simulink model "chap4_3sim"  (Simulink 5.0)
settings: Solver=ode45  StartTime=0.0  StopTime=20  RelTol=1e-5
settings Model: LastModifiedBy=Administrator  ExtModeTrigMode=oneshot  ExtModeArmWhenConnect=off  LimitDataPoints=off  BooleanDataType=off

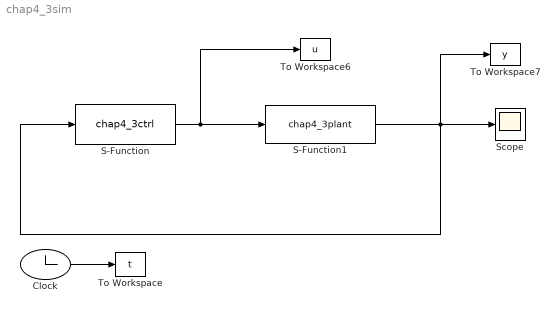
== system chap4_3sim ==
  Clock : Clock
  S-Function : S-Function  FunctionName=chap4_3ctrl
  S-Function1 : S-Function  FunctionName=chap4_3plant
  Scope : Scope
      settings: YMin=0.1  YMax=0.34
  To Workspace : ToWorkspace  VariableName=t  SampleTime=-1  SaveFormat=Array
  To Workspace6 : ToWorkspace  VariableName=u  SampleTime=-1  SaveFormat=Array
  To Workspace7 : ToWorkspace  VariableName=y  SampleTime=-1  SaveFormat=Array
  wires:
  S-Function/1 -> S-Function1/1, To Workspace6/1
  Clock/1 -> To Workspace/1
  S-Function1/1 -> S-Function/1, To Workspace7/1, Scope/1
